simulink model "ARCH_AT1_art"  (R2019b)
settings: Solver=FixedStepAuto  StartTime=0.0  StopTime=10.0  FixedStep=fixedStepSize  RelTol=1e-3
undefined symbols (not defined in the file): artificial_ARCH_AT1_max, artificial_ARCH_AT1_min, artificial_ARCH_AT1_time
settings Model: Creator=JEDDELAN  LastModifiedBy=JEDDELAN
settings DataIOCC: SaveOutput=off  SaveTime=off  ReturnWorkspaceOutputs=off
settings DebuggingCC: ArithmeticOperatorsInVariantConditions=warning
settings SFSimCC: SimUseLocalCustomCode=off  CustomCodeUndefinedFunction=UseInterfaceOnly
settings RTWCC: RTWUseLocalCustomCode=off
settings GRTTargetCC: CombineOutputUpdateFcns=off  MatFileLogging=off

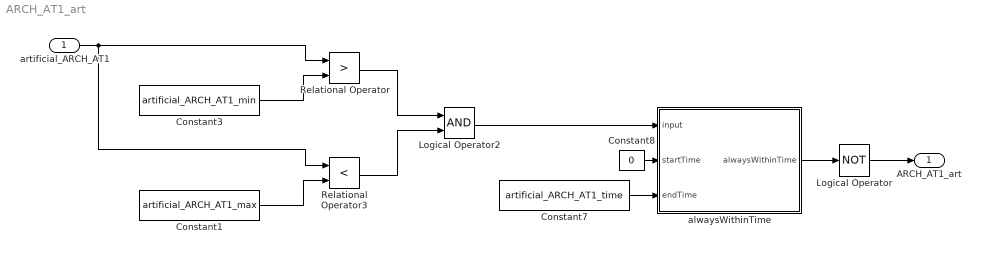
== system ARCH_AT1_art ==
  artificial_ARCH_AT1 : Inport
  Constant1 : Constant  Value=artificial_ARCH_AT1_max
  Constant3 : Constant  Value=artificial_ARCH_AT1_min
  Constant7 : Constant  Value=artificial_ARCH_AT1_time
  Constant8 : Constant  Value=0
  Logical Operator : Logic  Operator=NOT  AllPortsSameDT=off  OutDataTypeStr=boolean
  Logical Operator2 : Logic  AllPortsSameDT=off  OutDataTypeStr=boolean
  Relational Operator : RelationalOperator  Operator=>  OutDataTypeStr=boolean  RndMeth=Simplest
  Relational Operator3 : RelationalOperator  Operator=<  OutDataTypeStr=boolean  RndMeth=Simplest
  alwaysWithinTime : Subsystem
      settings: CopyFcn=set_param(gcbh,'LinkStatus','none');
  ARCH_AT1_art : Outport  OutDataTypeStr=boolean  PortDimensions=1  VectorParamsAs1DForOutWhenUnconnected=off
  wires:
  artificial_ARCH_AT1/1 -> Relational Operator3/1, Relational Operator/1
  Relational Operator/1 -> Logical Operator2/1
  Relational Operator3/1 -> Logical Operator2/2
  alwaysWithinTime/1(alwaysWithinTime) -> Logical Operator/1
  Constant7/1 -> alwaysWithinTime/3(endTime)
  Constant1/1 -> Relational Operator3/2
  Constant8/1 -> alwaysWithinTime/2(startTime)
  Logical Operator2/1 -> alwaysWithinTime/1(input)
  Constant3/1 -> Relational Operator/2
  Logical Operator/1 -> ARCH_AT1_art/1

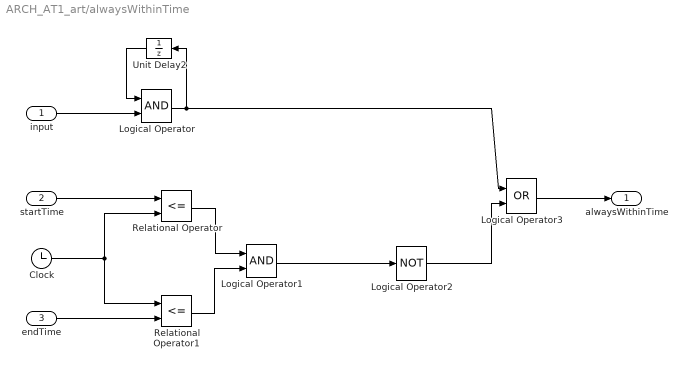
== system ARCH_AT1_art/alwaysWithinTime ==
  input : Inport
  startTime : Inport  Port=2
  endTime : Inport  Port=3
  Clock : Clock
  Logical Operator : Logic  AllPortsSameDT=off  OutDataTypeStr=boolean
  Logical Operator1 : Logic  AllPortsSameDT=off  OutDataTypeStr=boolean
  Logical Operator2 : Logic  Operator=NOT  AllPortsSameDT=off  OutDataTypeStr=boolean
  Logical Operator3 : Logic  Operator=OR  AllPortsSameDT=off  OutDataTypeStr=boolean
  Relational Operator : RelationalOperator  Operator=<=  OutDataTypeStr=boolean  RndMeth=Simplest
  Relational Operator1 : RelationalOperator  Operator=<=  OutDataTypeStr=boolean  RndMeth=Simplest
  Unit Delay2 : UnitDelay  InitialCondition=1  SampleTime=-1  HasFrameUpgradeWarning=on
  alwaysWithinTime : Outport  VectorParamsAs1DForOutWhenUnconnected=off
  wires:
  startTime/1 -> Relational Operator/1
  Unit Delay2/1 -> Logical Operator/1
  input/1 -> Logical Operator/2
  Logical Operator/1 -> Logical Operator3/1, Unit Delay2/1
  Clock/1 -> Relational Operator1/1, Relational Operator/2
  endTime/1 -> Relational Operator1/2
  Relational Operator1/1 -> Logical Operator1/2
  Relational Operator/1 -> Logical Operator1/1
  Logical Operator1/1 -> Logical Operator2/1
  Logical Operator2/1 -> Logical Operator3/2
  Logical Operator3/1 -> alwaysWithinTime/1
